simulink model "bms_slave"  (R2024b)
settings: Solver=ode4  StartTime=0.0  StopTime=T_stop  FixedStep=0.1  RelTol=1e-3
undefined symbols (not defined in the file): bms
libraries: simulink x13
settings Model: DataDictionary=buses.sldd  Creator=rayen  LastModifiedBy=rayen
settings OptimizationCC: DefaultParameterBehavior=Inlined  EnhancedBackFolding=on  PassReuseOutputArgsAs=Individual arguments  OptimizeBlockOrder=speed  DifferentSizesBufferReuse=on  OptimizationCustomize=off  EfficientTunableParamExpr=on
settings DebuggingCC: AlgebraicLoopMsg=error  ParameterTunabilityLossMsg=error
settings SFSimCC: MATLABDynamicMemAlloc=off
settings RTWCC: Description=Embedded Coder  SystemTargetFile=ert.tlc  TemplateMakefile=ert_default_tmf
settings CodeAppCC: ForceParamTrailComments=on  IgnoreCustomStorageClasses=off  OperatorAnnotations=on  SimulinkDataObjDesc=on  SFDataObjDesc=on  InsertBlockDesc=on
settings ERTTargetCC: TargetLangStandard=C99 (ISO)  GenerateSampleERTMain=on  CodeInterfacePackaging=Reusable function  ERTCustomFileTemplate=example_file_process.tlc

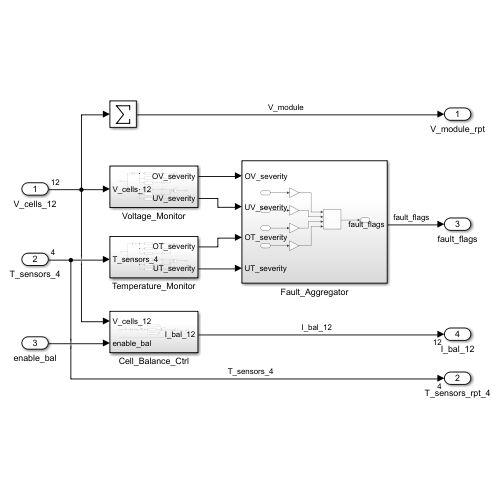
[thumbnail: Simulink's stored preview of the top-level diagram]
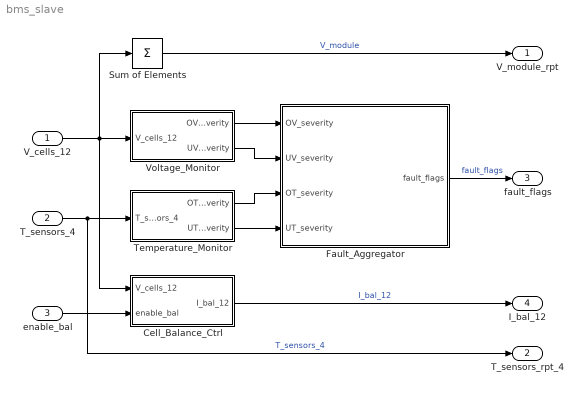
== system bms_slave ==
  V_cells_12 : Inport  OutDataTypeStr=double  PortDimensions=[12]
  T_sensors_4 : Inport  Port=2  OutDataTypeStr=double  PortDimensions=[4]
  enable_bal : Inport  Port=3  OutDataTypeStr=double  PortDimensions=1
  Cell_Balance_Ctrl : Subsystem
  Fault_Aggregator : Subsystem
  Sum of Elements : Sum  Inputs=+
  Temperature_Monitor : Subsystem
  Voltage_Monitor : Subsystem
  V_module_rpt : Outport  OutDataTypeStr=double  PortDimensions=1
  T_sensors_rpt_4 : Outport  Port=2  OutDataTypeStr=double  PortDimensions=[4]
  fault_flags : Outport  Port=3  OutDataTypeStr=double  PortDimensions=1
  I_bal_12 : Outport  Port=4  OutDataTypeStr=double  PortDimensions=[12]
  wires:
  Voltage_Monitor/1(OV_severity) -> Fault_Aggregator/1(OV_severity)
  Temperature_Monitor/2(UT_severity) -> Fault_Aggregator/4(UT_severity)
  Voltage_Monitor/2(UV_severity) -> Fault_Aggregator/2(UV_severity)
  Temperature_Monitor/1(OT_severity) -> Fault_Aggregator/3(OT_severity)
  T_sensors_4/1 -> T_sensors_rpt_4/1, Temperature_Monitor/1(T_sensors_4)  "T_sensors_4"
  V_cells_12/1 -> Sum of Elements/1, Voltage_Monitor/1(V_cells_12), Cell_Balance_Ctrl/1(V_cells_12)
  enable_bal/1 -> Cell_Balance_Ctrl/2(enable_bal)
  Cell_Balance_Ctrl/1(I_bal_12) -> I_bal_12/1  "I_bal_12"
  Fault_Aggregator/1(fault_flags) -> fault_flags/1  "fault_flags"
  Sum of Elements/1 -> V_module_rpt/1  "V_module"

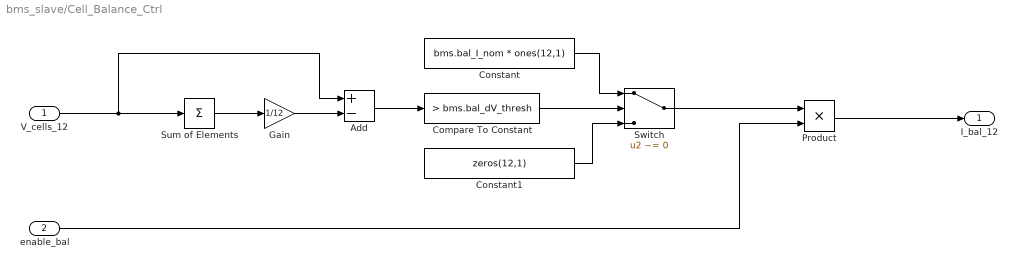
== system bms_slave/Cell_Balance_Ctrl ==
  V_cells_12 : Inport
  enable_bal : Inport  Port=2
  Add : Sum  Inputs=+-
  Compare To Constant : simulink/Logic and Bit Operations/Compare To Constant  relop=>  const=bms.bal_dV_thresh  OutDataTypeStr=boolean
  Constant : Constant  Value=bms.bal_I_nom * ones(12,1)
  Constant1 : Constant  Value=zeros(12,1)
  Gain : Gain  Gain=1/12
  Product : Product  OutDataTypeStr=double
  Sum of Elements : Sum  Inputs=+
  Switch : Switch  Criteria=u2 ~= 0  SaturateOnIntegerOverflow=off  InputSameDT=off
  I_bal_12 : Outport
  wires:
  Sum of Elements/1 -> Gain/1
  V_cells_12/1 -> Add/1, Sum of Elements/1
  Add/1 -> Compare To Constant/1
  Gain/1 -> Add/2
  Compare To Constant/1 -> Switch/2
  Constant/1 -> Switch/1
  Constant1/1 -> Switch/3
  Switch/1 -> Product/1
  Product/1 -> I_bal_12/1
  enable_bal/1 -> Product/2

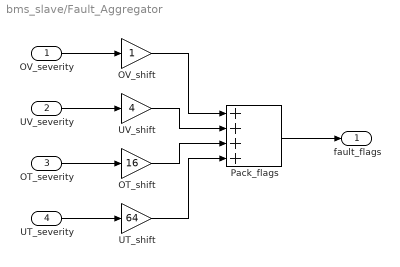
== system bms_slave/Fault_Aggregator ==
  OV_severity : Inport
  UV_severity : Inport  Port=2
  OT_severity : Inport  Port=3
  UT_severity : Inport  Port=4
  OT_shift : Gain  Gain=16  OutDataTypeStr=double
  OV_shift : Gain  OutDataTypeStr=double
  Pack_flags : Sum  Inputs=++++  OutDataTypeStr=double
  UT_shift : Gain  Gain=64  OutDataTypeStr=double
  UV_shift : Gain  Gain=4  OutDataTypeStr=double
  fault_flags : Outport
  wires:
  OV_severity/1 -> OV_shift/1
  UV_severity/1 -> UV_shift/1
  OT_severity/1 -> OT_shift/1
  UT_severity/1 -> UT_shift/1
  OV_shift/1 -> Pack_flags/1
  Pack_flags/1 -> fault_flags/1
  UT_shift/1 -> Pack_flags/4
  UV_shift/1 -> Pack_flags/2
  OT_shift/1 -> Pack_flags/3

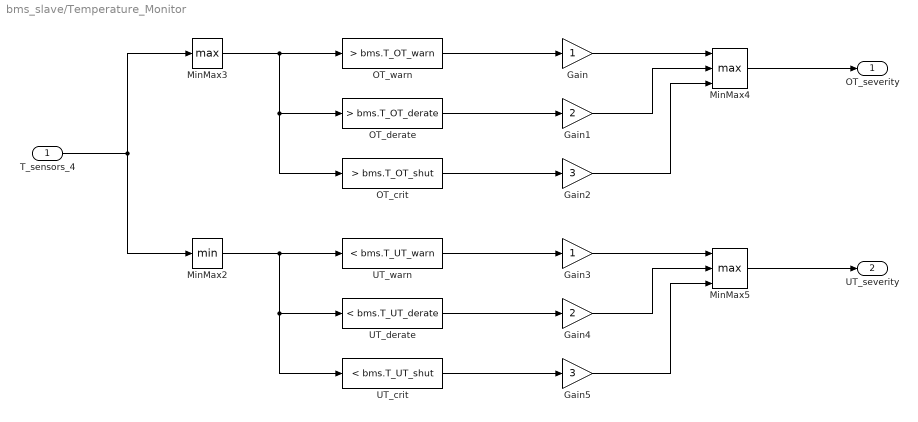
== system bms_slave/Temperature_Monitor ==
  T_sensors_4 : Inport
  Gain : Gain
  Gain1 : Gain  Gain=2
  Gain2 : Gain  Gain=3
  Gain3 : Gain
  Gain4 : Gain  Gain=2
  Gain5 : Gain  Gain=3
  MinMax2 : MinMax
  MinMax3 : MinMax  Function=max
  MinMax4 : MinMax  Function=max  Inputs=3
  MinMax5 : MinMax  Function=max  Inputs=3
  OT_crit : simulink/Logic and Bit Operations/Compare To Constant  relop=>  const=bms.T_OT_shut  OutDataTypeStr=boolean
  OT_derate : simulink/Logic and Bit Operations/Compare To Constant  relop=>  const=bms.T_OT_derate  OutDataTypeStr=boolean
  OT_warn : simulink/Logic and Bit Operations/Compare To Constant  relop=>  const=bms.T_OT_warn  OutDataTypeStr=boolean
  UT_crit : simulink/Logic and Bit Operations/Compare To Constant  relop=<  const=bms.T_UT_shut  OutDataTypeStr=boolean
  UT_derate : simulink/Logic and Bit Operations/Compare To Constant  relop=<  const=bms.T_UT_derate  OutDataTypeStr=boolean
  UT_warn : simulink/Logic and Bit Operations/Compare To Constant  relop=<  const=bms.T_UT_warn  OutDataTypeStr=boolean
  OT_severity : Outport
  UT_severity : Outport  Port=2
  wires:
  UT_warn/1 -> Gain3/1
  Gain/1 -> MinMax4/1
  OT_crit/1 -> Gain2/1
  UT_derate/1 -> Gain4/1
  UT_crit/1 -> Gain5/1
  Gain5/1 -> MinMax5/3
  Gain3/1 -> MinMax5/1
  MinMax4/1 -> OT_severity/1
  Gain4/1 -> MinMax5/2
  OT_derate/1 -> Gain1/1
  Gain2/1 -> MinMax4/3
  T_sensors_4/1 -> MinMax2/1, MinMax3/1
  OT_warn/1 -> Gain/1
  MinMax3/1 -> OT_crit/1, OT_derate/1, OT_warn/1
  Gain1/1 -> MinMax4/2
  MinMax2/1 -> UT_derate/1, UT_crit/1, UT_warn/1
  MinMax5/1 -> UT_severity/1

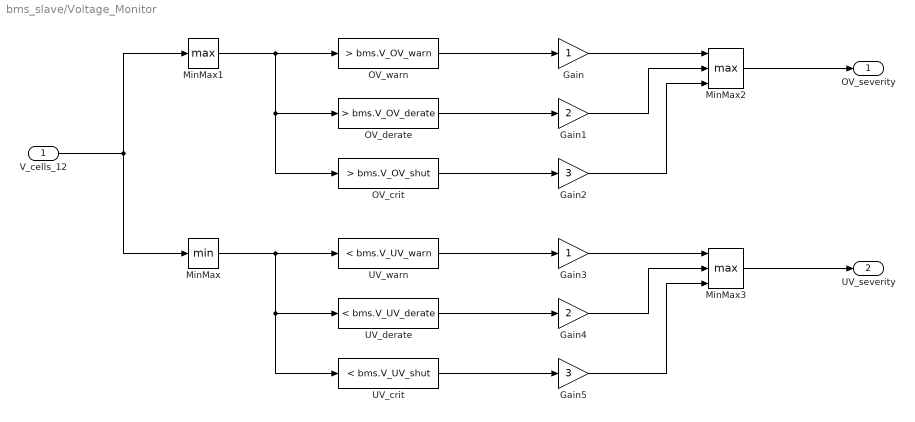
== system bms_slave/Voltage_Monitor ==
  V_cells_12 : Inport
  Gain : Gain
  Gain1 : Gain  Gain=2
  Gain2 : Gain  Gain=3
  Gain3 : Gain
  Gain4 : Gain  Gain=2
  Gain5 : Gain  Gain=3
  MinMax : MinMax
  MinMax1 : MinMax  Function=max
  MinMax2 : MinMax  Function=max  Inputs=3
  MinMax3 : MinMax  Function=max  Inputs=3
  OV_crit : simulink/Logic and Bit Operations/Compare To Constant  relop=>  const=bms.V_OV_shut  OutDataTypeStr=boolean
  OV_derate : simulink/Logic and Bit Operations/Compare To Constant  relop=>  const=bms.V_OV_derate  OutDataTypeStr=boolean
  OV_warn : simulink/Logic and Bit Operations/Compare To Constant  relop=>  const=bms.V_OV_warn  OutDataTypeStr=boolean
  UV_crit : simulink/Logic and Bit Operations/Compare To Constant  relop=<  const=bms.V_UV_shut  OutDataTypeStr=boolean
  UV_derate : simulink/Logic and Bit Operations/Compare To Constant  relop=<  const=bms.V_UV_derate  OutDataTypeStr=boolean
  UV_warn : simulink/Logic and Bit Operations/Compare To Constant  relop=<  const=bms.V_UV_warn  OutDataTypeStr=boolean
  OV_severity : Outport
  UV_severity : Outport  Port=2
  wires:
  V_cells_12/1 -> MinMax/1, MinMax1/1
  MinMax1/1 -> OV_crit/1, OV_derate/1, OV_warn/1
  MinMax/1 -> UV_derate/1, UV_crit/1, UV_warn/1
  OV_warn/1 -> Gain/1
  Gain/1 -> MinMax2/1
  OV_derate/1 -> Gain1/1
  OV_crit/1 -> Gain2/1
  Gain1/1 -> MinMax2/2
  Gain2/1 -> MinMax2/3
  Gain3/1 -> MinMax3/1
  UV_crit/1 -> Gain5/1
  UV_derate/1 -> Gain4/1
  Gain4/1 -> MinMax3/2
  Gain5/1 -> MinMax3/3
  UV_warn/1 -> Gain3/1
  MinMax3/1 -> UV_severity/1
  MinMax2/1 -> OV_severity/1
